simulink model "fp_model"  (R2024a)
settings: Solver=FixedStepAuto  StartTime=0.0  StopTime=10.0  RelTol=1e-3
values from neighbouring files (symbols this model uses):
  buffer_size = 512    [workspace.mat]
  sampling_freq = 29900    [workspace.mat]
libraries: dspxfrm3 x1
settings Model: Creator=Jan Rosa  LastModifiedBy=Jan Rosa

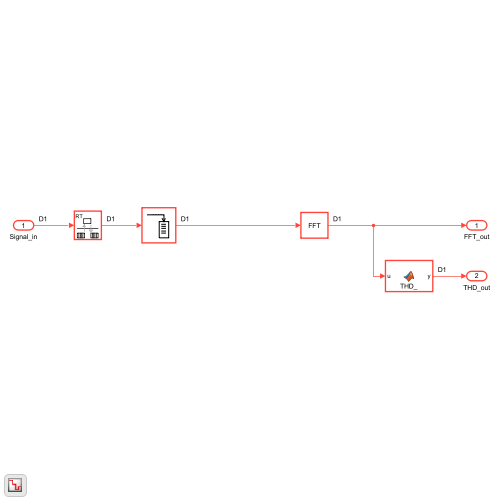
[thumbnail: Simulink's stored preview of the top-level diagram]
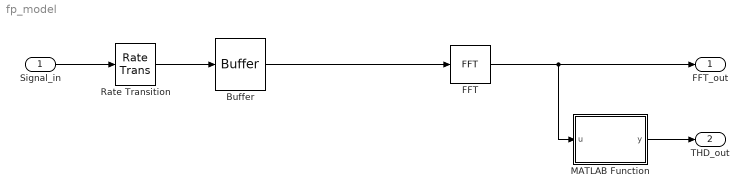
== system fp_model ==
  Signal_in : Inport
  Buffer : Buffer  N=buffer_size  V=buffer_size-1  OutputFrames=off
  FFT : dspxfrm3/FFT  FFTImplementation=Auto  CompMethod=Table lookup  TableOpt=NEW  TableOptActive=Speed  BitRevOrder=off  Normalize=on  InheritFFTLength=on  FFTLength=64  WrapInput=on  roundingMode=Ceiling  overflowMode=off  firstCoeffDataTypeStr=Inherit: Same word length as input  firstCoeffLastDataTypeStr=Inherit: Same word length as input  outputMin=[]  outputMax=[]
  MATLAB Function : MATLAB Function  TreatAsAtomicUnit=on
  Rate Transition : RateTransition  OutPortSampleTime=1/sampling_freq
  FFT_out : Outport
  THD_out : Outport  Port=2
  wires:
  Buffer/1 -> FFT/1
  FFT/1 -> MATLAB Function/1(u), FFT_out/1
  MATLAB Function/1(y) -> THD_out/1
  Signal_in/1 -> Rate Transition/1
  Rate Transition/1 -> Buffer/1

== matlab function fp_model/MATLAB Function ==
  data: u input; y output
function y = THD_(u)

y = abs( rms(abs(u(2:end))) / abs(u(1)) );
